simulink model "SVPWM"  (R2018b)
settings: Solver=ode23tb  StartTime=0.0  StopTime=10.0  MaxStep=0.00001  RelTol=1e-3
libraries: simulink x1
settings Model: Creator=Lenovo  LastModifiedBy=Lenovo

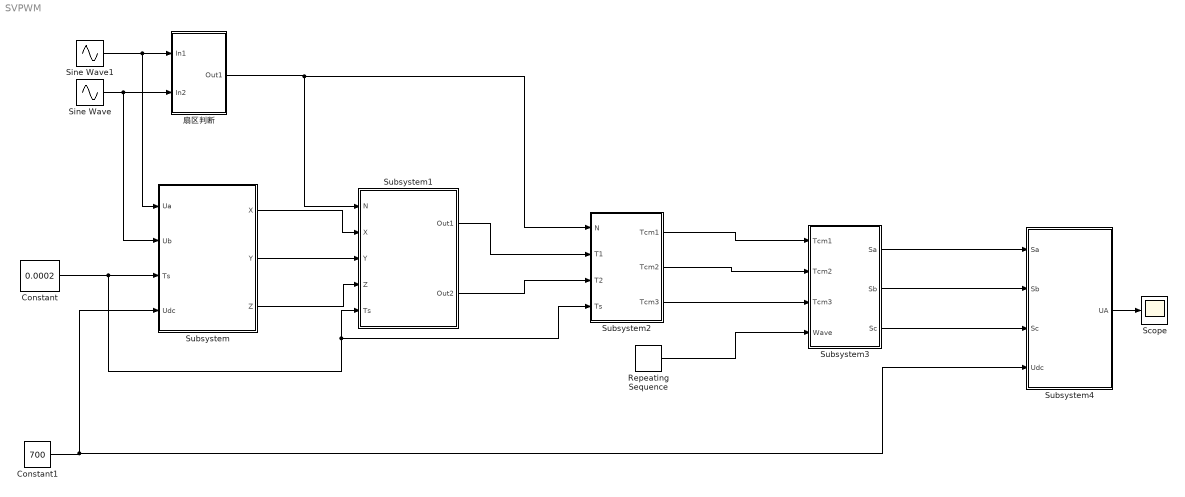
== system SVPWM ==
  Constant : Constant  Value=0.0002
  Constant1 : Constant  Value=700
  Repeating Sequence : simulink/Sources/Repeating Sequence  rep_seq_t=[0 1/10000 1/5000]  rep_seq_y=[0 1/10000 0]
  Scope : Scope
  Sine Wave : Sin  Amplitude=200  Frequency=100*pi  SampleTime=0
  Sine Wave1 : Sin  Amplitude=200  Frequency=100*pi  Phase=pi/2  SampleTime=0
  Subsystem : Subsystem
  Subsystem1 : Subsystem
      mask Display:
      | port_label('output' , 1 , 'T1');
      | port_label('output' , 2 , 'T2');
      | port_label('input' , 1 , 'N');
      | port_label('input' , 2 , 'X');
      | port_label('input' , 3 , 'Y');
      | port_label('input' , 4 , 'Z');
      | port_label('input' , 5 , 'Ts');
  Subsystem2 : Subsystem
  Subsystem3 : Subsystem
  Subsystem4 : Subsystem
  扇区判断 : Subsystem
      mask Display:
      | port_label('input' , 1 , 'Ua');
      | port_label('input' , 2 , 'Ub');
      | port_label('output' , 1 , 'N');
  wires:
  Sine Wave/1 -> Subsystem/2(Ub), 扇区判断/2(In2)
  Sine Wave1/1 -> Subsystem/1(Ua), 扇区判断/1(In1)
  Constant/1 -> Subsystem2/4(Ts), Subsystem1/5(Ts), Subsystem/3(Ts)
  Constant1/1 -> Subsystem4/4(Udc), Subsystem/4(Udc)
  扇区判断/1(Out1) -> Subsystem2/1(N), Subsystem1/1(N)
  Subsystem/1(X) -> Subsystem1/2(X)
  Subsystem/2(Y) -> Subsystem1/3(Y)
  Subsystem/3(Z) -> Subsystem1/4(Z)
  Subsystem1/1(Out1) -> Subsystem2/2(T1)
  Subsystem1/2(Out2) -> Subsystem2/3(T2)
  Repeating Sequence/1 -> Subsystem3/4(Wave)
  Subsystem2/3(Tcm3) -> Subsystem3/3(Tcm3)
  Subsystem2/2(Tcm2) -> Subsystem3/2(Tcm2)
  Subsystem2/1(Tcm1) -> Subsystem3/1(Tcm1)
  Subsystem3/1(Sa) -> Subsystem4/1(Sa)
  Subsystem3/2(Sb) -> Subsystem4/2(Sb)
  Subsystem3/3(Sc) -> Subsystem4/3(Sc)
  Subsystem4/1(UA) -> Scope/1

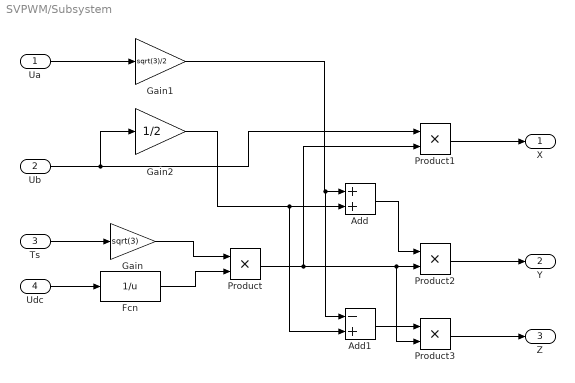
== system SVPWM/Subsystem ==
  Ua : Inport
  Ub : Inport  Port=2
  Ts : Inport  Port=3
  Udc : Inport  Port=4
  Add : Sum
  Add1 : Sum  Inputs=-+
  Fcn : Fcn  Expr=1/u
  Gain : Gain  Gain=sqrt(3)
  Gain1 : Gain  Gain=sqrt(3)/2
  Gain2 : Gain  Gain=1/2
  Product{,1..3} (4 alike) : Product
  X : Outport
  Y : Outport  Port=2
  Z : Outport  Port=3
  wires:
  Product2/1 -> Y/1
  Product/1 -> Product3/2, Product2/2, Product1/2
  Product1/1 -> X/1
  Fcn/1 -> Product/2
  Ts/1 -> Gain/1
  Gain1/1 -> Add1/1, Add/1
  Product3/1 -> Z/1
  Add/1 -> Product2/1
  Ua/1 -> Gain1/1
  Ub/1 -> Gain2/1, Product1/1
  Add1/1 -> Product3/1
  Gain2/1 -> Add1/2, Add/2
  Udc/1 -> Fcn/1
  Gain/1 -> Product/1

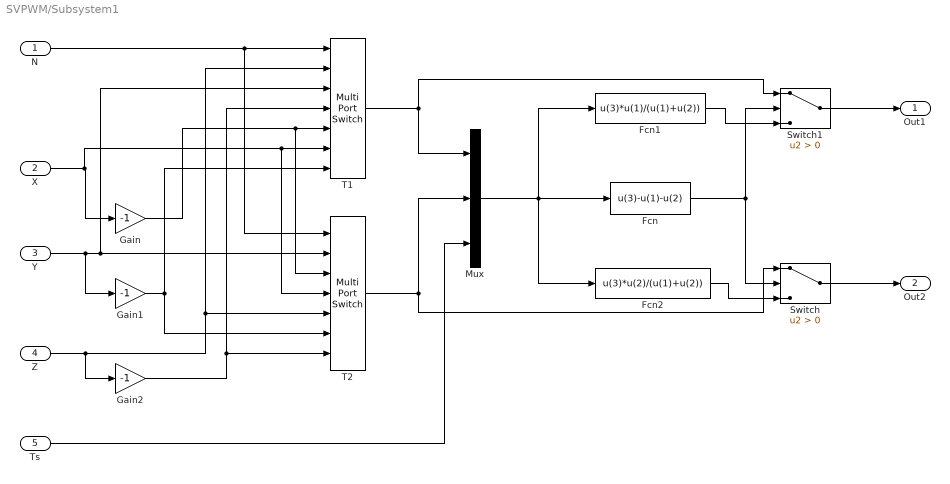
== system SVPWM/Subsystem1 ==
  N : Inport
  X : Inport  Port=2
  Y : Inport  Port=3
  Z : Inport  Port=4
  Ts : Inport  Port=5
  Fcn : Fcn  Expr=u(3)-u(1)-u(2)
  Fcn1 : Fcn  Expr=u(3)*u(1)/(u(1)+u(2))
  Fcn2 : Fcn  Expr=u(3)*u(2)/(u(1)+u(2))
  Gain : Gain  Gain=-1
  Gain1 : Gain  Gain=-1
  Gain2 : Gain  Gain=-1
  Mux : Mux  Inputs=3
  Switch : Switch  Criteria=u2 > Threshold
  Switch1 : Switch  Criteria=u2 > Threshold
  T1 : MultiPortSwitch  Inputs=6
  T2 : MultiPortSwitch  Inputs=6
  Out1 : Outport
  Out2 : Outport  Port=2
  wires:
  Fcn1/1 -> Switch1/3
  T2/1 -> Mux/2, Switch/1
  N/1 -> T2/1, T1/1
  Mux/1 -> Fcn/1, Fcn2/1, Fcn1/1
  X/1 -> T2/4, T1/6, Gain/1
  Y/1 -> T2/2, T1/3, Gain1/1
  Gain/1 -> T2/3, T1/5
  T1/1 -> Mux/1, Switch1/1
  Z/1 -> T2/5, T1/2, Gain2/1
  Gain2/1 -> T2/7, T1/4
  Switch1/1 -> Out1/1
  Fcn/1 -> Switch/2, Switch1/2
  Gain1/1 -> T2/6, T1/7
  Switch/1 -> Out2/1
  Ts/1 -> Mux/3
  Fcn2/1 -> Switch/3

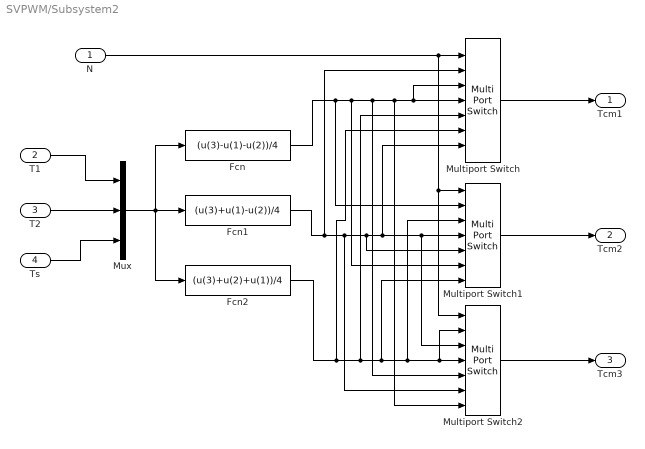
== system SVPWM/Subsystem2 ==
  N : Inport
  T1 : Inport  Port=2
  T2 : Inport  Port=3
  Ts : Inport  Port=4
  Fcn : Fcn  Expr=(u(3)-u(1)-u(2))/4
  Fcn1 : Fcn  Expr=(u(3)+u(1)-u(2))/4
  Fcn2 : Fcn  Expr=(u(3)+u(2)+u(1))/4
  Multiport Switch : MultiPortSwitch  Inputs=6
  Multiport Switch1 : MultiPortSwitch  Inputs=6
  Multiport Switch2 : MultiPortSwitch  Inputs=6
  Mux : Mux  Inputs=3
  Tcm1 : Outport
  Tcm2 : Outport  Port=2
  Tcm3 : Outport  Port=3
  wires:
  Ts/1 -> Mux/3
  T1/1 -> Mux/1
  Mux/1 -> Fcn/1, Fcn2/1, Fcn1/1
  T2/1 -> Mux/2
  Multiport Switch1/1 -> Tcm2/1
  Multiport Switch/1 -> Tcm1/1
  Multiport Switch2/1 -> Tcm3/1
  N/1 -> Multiport Switch/1, Multiport Switch1/1, Multiport Switch2/1
  Fcn/1 -> Multiport Switch1/2, Multiport Switch1/6, Multiport Switch2/5, Multiport Switch2/7, Multiport Switch/3, Multiport Switch/4
  Fcn1/1 -> Multiport Switch/2, Multiport Switch2/6, Multiport Switch1/5, Multiport Switch/7, Multiport Switch2/3, Multiport Switch1/4
  Fcn2/1 -> Multiport Switch/6, Multiport Switch/5, Multiport Switch1/7, Multiport Switch1/3, Multiport Switch2/2, Multiport Switch2/4

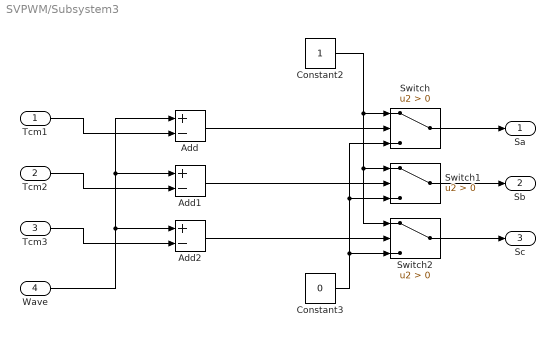
== system SVPWM/Subsystem3 ==
  Tcm1 : Inport
  Tcm2 : Inport  Port=2
  Tcm3 : Inport  Port=3
  Wave : Inport  Port=4
  Add : Sum  Inputs=+-
  Add1 : Sum  Inputs=+-
  Add2 : Sum  Inputs=+-
  Constant2 : Constant
  Constant3 : Constant  Value=0
  Switch : Switch  Criteria=u2 > Threshold
  Switch1 : Switch  Criteria=u2 > Threshold
  Switch2 : Switch  Criteria=u2 > Threshold
  Sa : Outport
  Sb : Outport  Port=2
  Sc : Outport  Port=3
  wires:
  Constant3/1 -> Switch2/3, Switch1/3, Switch/3
  Add1/1 -> Switch1/2
  Switch2/1 -> Sc/1
  Add/1 -> Switch/2
  Constant2/1 -> Switch2/1, Switch1/1, Switch/1
  Tcm1/1 -> Add/2
  Wave/1 -> Add2/1, Add1/1, Add/1
  Switch1/1 -> Sb/1
  Add2/1 -> Switch2/2
  Switch/1 -> Sa/1
  Tcm2/1 -> Add1/2
  Tcm3/1 -> Add2/2

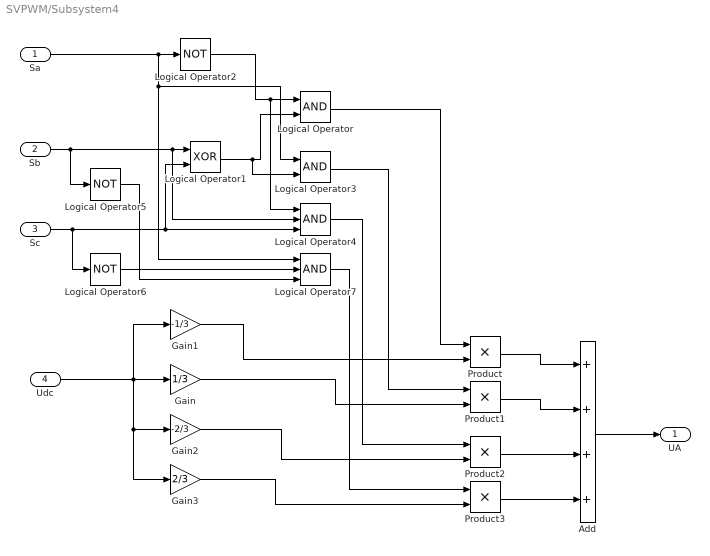
== system SVPWM/Subsystem4 ==
  Sa : Inport
  Sb : Inport  Port=2
  Sc : Inport  Port=3
  Udc : Inport  Port=4
  Add : Sum  Inputs=++++
  Gain : Gain  Gain=1/3
  Gain1 : Gain  Gain=-1/3
  Gain2 : Gain  Gain=-2/3
  Gain3 : Gain  Gain=2/3
  Logical Operator : Logic  AllPortsSameDT=off  OutDataTypeStr=boolean
  Logical Operator1 : Logic  Operator=XOR  AllPortsSameDT=off  OutDataTypeStr=boolean
  Logical Operator2 : Logic  Operator=NOT  AllPortsSameDT=off  OutDataTypeStr=boolean
  Logical Operator3 : Logic  AllPortsSameDT=off  OutDataTypeStr=boolean
  Logical Operator4 : Logic  Inputs=3  AllPortsSameDT=off  OutDataTypeStr=boolean
  Logical Operator5 : Logic  Operator=NOT  AllPortsSameDT=off  OutDataTypeStr=boolean
  Logical Operator6 : Logic  Operator=NOT  AllPortsSameDT=off  OutDataTypeStr=boolean
  Logical Operator7 : Logic  Inputs=3  AllPortsSameDT=off  OutDataTypeStr=boolean
  Product{,1..3} (4 alike) : Product
  UA : Outport
  wires:
  Sc/1 -> Logical Operator6/1, Logical Operator4/3, Logical Operator1/2
  Gain/1 -> Product1/2
  Udc/1 -> Gain3/1, Gain2/1, Gain1/1, Gain/1
  Logical Operator3/1 -> Product1/1
  Gain1/1 -> Product/2
  Sb/1 -> Logical Operator5/1, Logical Operator4/2, Logical Operator1/1
  Logical Operator1/1 -> Logical Operator3/2, Logical Operator/2
  Logical Operator2/1 -> Logical Operator4/1, Logical Operator/1
  Logical Operator7/1 -> Product3/1
  Sa/1 -> Logical Operator7/1, Logical Operator3/1, Logical Operator2/1
  Gain2/1 -> Product2/2
  Add/1 -> UA/1
  Product/1 -> Add/1
  Logical Operator6/1 -> Logical Operator7/2
  Product1/1 -> Add/2
  Gain3/1 -> Product3/2
  Logical Operator/1 -> Product/1
  Product2/1 -> Add/3
  Product3/1 -> Add/4
  Logical Operator4/1 -> Product2/1
  Logical Operator5/1 -> Logical Operator7/3

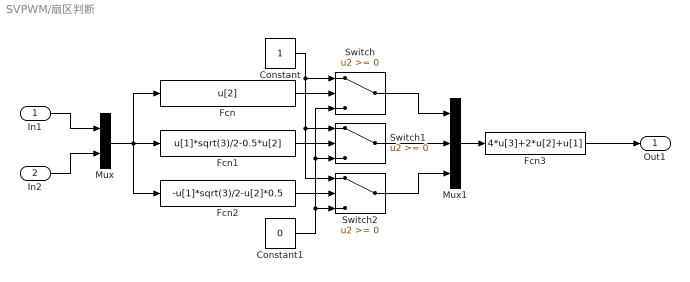
== system SVPWM/扇区判断 ==
  In1 : Inport
  In2 : Inport  Port=2
  Constant : Constant
  Constant1 : Constant  Value=0
  Fcn : Fcn  Expr=u[2]
  Fcn1 : Fcn  Expr=u[1]*sqrt(3)/2-0.5*u[2]
  Fcn2 : Fcn  Expr=-u[1]*sqrt(3)/2-u[2]*0.5
  Fcn3 : Fcn  Expr=4*u[3]+2*u[2]+u[1]
  Mux : Mux  Inputs=2
  Mux1 : Mux  Inputs=3
  Switch : Switch
  Switch1 : Switch
  Switch2 : Switch
  Out1 : Outport
  wires:
  Switch1/1 -> Mux1/2
  Constant1/1 -> Switch2/3, Switch/3, Switch1/3
  Fcn2/1 -> Switch2/2
  Mux1/1 -> Fcn3/1
  Constant/1 -> Switch/1, Switch2/1, Switch1/1
  Mux/1 -> Fcn2/1, Fcn/1, Fcn1/1
  In2/1 -> Mux/2
  In1/1 -> Mux/1
  Fcn3/1 -> Out1/1
  Switch/1 -> Mux1/1
  Fcn1/1 -> Switch1/2
  Fcn/1 -> Switch/2
  Switch2/1 -> Mux1/3
